simulink model "complete_controller_unorganized"  (R2023a)
settings: Solver=FixedStepAuto  StartTime=0.0  StopTime=inf  FixedStep=0.01  RelTol=1e-3
model workspace (MAT data in the model file):
  SL_ROS_VariableLengthArrays_MaxSizes.CommonInfo.ArrayTruncateAction = 'EmitWarning'
  SL_ROS_VariableLengthArrays_MaxSizes.MsgTypeMap = containers.Map
  SL_ROS_VariableLengthArrays_MaxSizes.MsgTypeMap.serialization.keys = {'diagnostic_msgs/DiagnosticArray', 'diagnostic_msgs/DiagnosticStatus', 'std_msgs/Float32MultiArray', 'std_msgs/Int32MultiArray'}
  SL_ROS_VariableLengthArrays_MaxSizes.MsgTypeMap.serialization.values{1}.PropertyName = 'status'
  SL_ROS_VariableLengthArrays_MaxSizes.MsgTypeMap.serialization.values{1}.DataType = 'diagnostic_msgs/DiagnosticStatus'
  SL_ROS_VariableLengthArrays_MaxSizes.MsgTypeMap.serialization.values{1}.MaxLength = 2
  SL_ROS_VariableLengthArrays_MaxSizes.MsgTypeMap.serialization.values{2}(1).PropertyName = 'hardware_id'
  SL_ROS_VariableLengthArrays_MaxSizes.MsgTypeMap.serialization.values{2}(1).DataType = 'uint8'
  SL_ROS_VariableLengthArrays_MaxSizes.MsgTypeMap.serialization.values{2}(1).MaxLength = 128
  SL_ROS_VariableLengthArrays_MaxSizes.MsgTypeMap.serialization.values{2}(2).PropertyName = 'message'
  SL_ROS_VariableLengthArrays_MaxSizes.MsgTypeMap.serialization.values{2}(2).DataType = 'uint8'
  SL_ROS_VariableLengthArrays_MaxSizes.MsgTypeMap.serialization.values{2}(2).MaxLength = 128
  SL_ROS_VariableLengthArrays_MaxSizes.MsgTypeMap.serialization.values{2}(3).PropertyName = 'name'
  SL_ROS_VariableLengthArrays_MaxSizes.MsgTypeMap.serialization.values{2}(3).DataType = 'uint8'
  SL_ROS_VariableLengthArrays_MaxSizes.MsgTypeMap.serialization.values{2}(3).MaxLength = 128
  SL_ROS_VariableLengthArrays_MaxSizes.MsgTypeMap.serialization.values{2}(4).PropertyName = 'values'
  SL_ROS_VariableLengthArrays_MaxSizes.MsgTypeMap.serialization.values{2}(4).DataType = 'diagnostic_msgs/KeyValue'
  SL_ROS_VariableLengthArrays_MaxSizes.MsgTypeMap.serialization.values{2}(4).MaxLength = 8
  SL_ROS_VariableLengthArrays_MaxSizes.MsgTypeMap.serialization.values{3}.PropertyName = 'data'
  SL_ROS_VariableLengthArrays_MaxSizes.MsgTypeMap.serialization.values{3}.DataType = 'single'
  SL_ROS_VariableLengthArrays_MaxSizes.MsgTypeMap.serialization.values{3}.MaxLength = 8
  SL_ROS_VariableLengthArrays_MaxSizes.MsgTypeMap.serialization.values{4}.PropertyName = 'data'
  SL_ROS_VariableLengthArrays_MaxSizes.MsgTypeMap.serialization.values{4}.DataType = 'int32'
  SL_ROS_VariableLengthArrays_MaxSizes.MsgTypeMap.serialization.values{4}.MaxLength = 8
  SL_ROS_VariableLengthArrays_MaxSizes.MsgTypeMap.serialization.uniformity = 0
  SL_ROS_VariableLengthArrays_MaxSizes.MsgTypeMap.serialization.keyType = 'char'
  SL_ROS_VariableLengthArrays_MaxSizes.MsgTypeMap.serialization.valueType = 'any'
undefined symbols (not defined in the file): angular, Btrigger_boost, DAapply_nudges, DAdesired_pose, DAff_body_force, DAsolver_weights, Djoy_R_X, Dreverse_throttle, Dthrottle, Iangular_mode, Ilinear_mode, linear
libraries: ros2lib x78
(part 1 of 3)
settings Model: Creator=hollis  LastModifiedBy=john
settings OptimizationCC: DefaultParameterBehavior=Inlined  GainParamInheritBuiltInType=on  UseFloatMulNetSlope=on  InlineInvariantSignals=on  EnhancedBackFolding=on  PassReuseOutputArgsAs=Individual arguments  ZeroExternalMemoryAtStartup=off  ZeroInternalMemoryAtStartup=off  EfficientFloat2IntCast=on  MaxStackSize=64  OptimizeBlockOrder=speed  DifferentSizesBufferReuse=on  OptimizationCustomize=off  EfficientTunableParamExpr=on
settings DebuggingCC: ParameterTunabilityLossMsg=error  UnderSpecifiedDimensionMsg=warning
settings HardwareCC: ProdBitPerLong=64  ProdLargestAtomicInteger=LongLong  ProdLargestAtomicFloat=Double  ProdLongLongMode=on  ProdHWDeviceType=ARM Compatible->ARM 64-bit (LP64)
settings SFSimCC: SimUserSources=complete_system/send_thruster_cmd_canbus.c  SimTargetLang=C++
settings RTWCC: Description=Embedded Coder  SystemTargetFile=ert.tlc  HardwareBoard=Robot Operating System 2 (ROS 2)  TLCOptions="-aInlineSetEventsForThisBaseRateFcn=TLC_FALSE -aSuppressMultiTaskScheduler=TLC_FALSE  -aRateBasedStepFcn=0"  TemplateMakefile=ert_default_tmf  CustomSource=complete_system/send_thruster_cmd_canbus.c  Toolchain=Colcon Tools  BuildConfiguration=Faster Runs  TargetLang=C++
settings CodeAppCC: ForceParamTrailComments=on  IgnoreCustomStorageClasses=off  OperatorAnnotations=on  SimulinkDataObjDesc=on  SFDataObjDesc=on  InsertBlockDesc=on
settings ERTTargetCC: TargetLangStandard=C++11 (ISO)  CodeInterfacePackaging=C++ class  SupportVariableSizeSignals=on  InlinedParameterPlacement=NonHierarchical  RootIOFormat=Structure reference

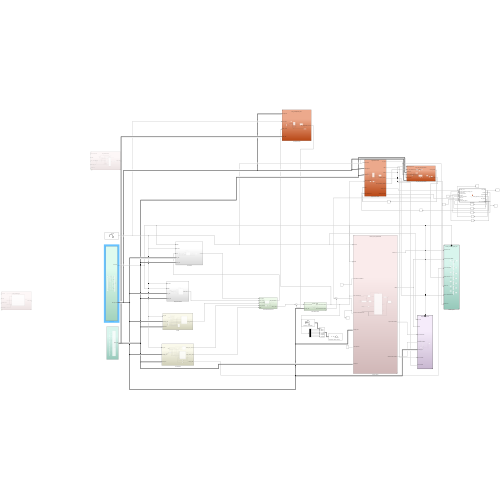
[thumbnail: Simulink's stored preview of the top-level diagram]
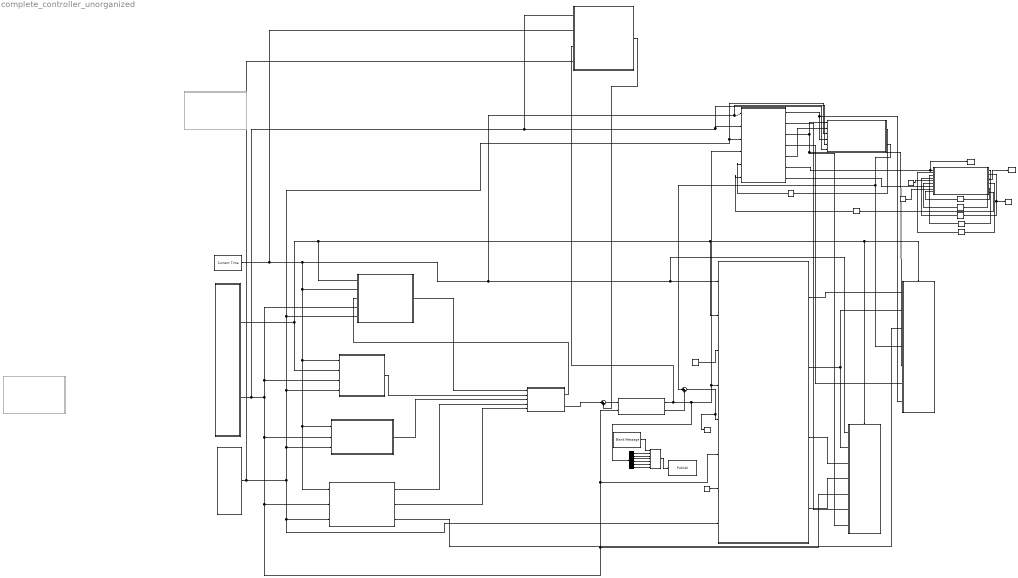
== system complete_controller_unorganized ==
  Applied Force Scale : Subsystem  ReferencedSubsystem=AppliedForceScale
  Auto_FF_Scale_Processor : Subsystem  ReferencedSubsystem=Auto_FF_Scale_Processor
  Blank Message : ros2lib/Blank Message  messageClass=Message  entityType=geometry_msgs/Twist  messageType=geometry_msgs/Twist  SampleTime=inf
  Bus Assignment : BusAssignment  AssignedSignals=linear.x,linear.y,linear.z,angular.x,angular.y,angular.z
  Constant : Constant
  Constant1 : Constant  Value=.005
  Constant2 : Constant  Value=15000
  Constant3 : Constant  Value=[0,0,0]
  Control Mask Management : Subsystem
  Control Mode Mask : Subsystem  ReferencedSubsystem=Disable_Gains
  Current Time : ros2lib/Current Time  OutputFormat=double  SampleTime=-1  ModelName=complete_controller
  Demux : Demux  Outputs=6
  Drag Compensator : Subsystem  ReferencedSubsystem=Drag_Compensator_mk1
  Memory : Memory  InitialCondition=false
  Memory1 : Memory  InitialCondition=[0;0;0]
  Memory2 : Memory
  Memory3 : Memory  InitialCondition=[0;0;0;0;0;0]
  Memory4 : Memory
  Memory5 : Memory
  Memory6 : Memory  InitialCondition=false
  PID Control2 : Subsystem
  Publish : ros2lib/Publish  topicSource=Specify your own  topic=/talos/controller_debug_wrench  messageType=geometry_msgs/Twist  QOSHistory=Keep last  QOSDepth=1  QOSReliability=Reliable  QOSDurability=Volatile
  Publish System : Subsystem  ReferencedSubsystem=Publish_Control_System_Out
  Record : Record  FileSettingsInternal="{\"entries\":[{\"content\":{\"excelSettings\":{\"content\":{},\"type\":\"Streamout.ExcelSettings\"}},\"type\":\"Streamout.FileSettingStorage\",\"uuid\":\"\"}],\"packageUris\":[\"http:\\/\\/schema.mathworks.com\\/mf0\\/streamout_blocks\\/R2020a\"],\"version\":\"1.0\"}"  Layout=[1 1]  SignalsInternal="{\"entries\":[{\"content\":{\"signals\":[{\"content\":{\"blockPath\":[],\"dimensions\":[6,1],\"domain\":\"\",\"hasChildren\":true,\"lineColor\":\"#4dbeee\",\"port\":1,\"signalID\":48,\"signalName\":\"com learner:2\"},\"type\":\"RecordBlkView.Signal\",\"uuid\":\"\"},{\"content\":{\"blockPath\":[],\"channel\":[1,1],\"dimensions\":[6,1],\"domain\":\"\",\"lineColor\":\"#ff13a6\",\"parentID\":48,\"port\":1,\"signalID\":49,\"signalName\":\"com learner:2\"},\"type\":\"RecordBlkView.Signal\",\"uuid\":\"\"}]},\"type\":\"RecordBlkView.InputSignals\",\"uuid\":\"\"}],\"packageUris\":[\"http:\\/\\/schema.mathworks.com\\/mf0\\/streamout_blocks\\/R2020a\"],\"version\":\"1.0\"}"  VisualizationBindings="{\"sparklinesplugin\":{\"info\":[{\"bindingParametersList\":[],\"subplotID\":1}]}}"
  Record1 : Record  FileSettingsInternal="{\"entries\":[{\"content\":{\"excelSettings\":{\"content\":{},\"type\":\"Streamout.ExcelSettings\"}},\"type\":\"Streamout.FileSettingStorage\",\"uuid\":\"\"}],\"packageUris\":[\"http:\\/\\/schema.mathworks.com\\/mf0\\/streamout_blocks\\/R2020a\"],\"version\":\"1.0\"}"  Layout=[1 1]  SignalsInternal="{\"entries\":[{\"content\":{\"signals\":[{\"content\":{\"blockPath\":[],\"dimensions\":[6,1],\"domain\":\"\",\"hasChildren\":true,\"lineColor\":\"#139fff\",\"port\":1,\"signalID\":36,\"signalName\":\"Applied Force Scale:6\"},\"type\":\"RecordBlkView.Signal\",\"uuid\":\"\"},{\"content\":{\"blockPath\":[],\"channel\":[1,1],\"dimensions\":[6,1],\"domain\":\"\",\"lineColor\":\"#22b573\",\"parentID\":36,\"port\":1,\"signalID\":37,\"signalName\":\"Applied Force Scale:6\"},\"type\":\"RecordBlkView.Signal\",\"uuid\":\"\"}]},\"type\":\"RecordBlkView.InputSignals\",\"uuid\":\"\"}],\"packageUris\":[\"http:\\/\\/schema.mathworks.com\\/mf0\\/streamout_blocks\\/R2020a\"],\"version\":\"1.0\"}"  VisualizationBindings="{\"sparklinesplugin\":{\"info\":[{\"bindingParametersList\":[],\"subplotID\":1}]}}"
  Record2 : Record  FileSettingsInternal="{\"entries\":[{\"content\":{\"excelSettings\":{\"content\":{},\"type\":\"Streamout.ExcelSettings\"}},\"type\":\"Streamout.FileSettingStorage\",\"uuid\":\"\"}],\"packageUris\":[\"http:\\/\\/schema.mathworks.com\\/mf0\\/streamout_blocks\\/R2020a\"],\"version\":\"1.0\"}"  SignalsInternal="{\"entries\":[{\"content\":{\"signals\":[{\"content\":{\"blockPath\":[],\"dimensions\":[3,1],\"domain\":\"\",\"hasChildren\":true,\"lineColor\":\"#b746ff\",\"port\":1,\"signalID\":25,\"signalName\":\"com learner:3\"},\"type\":\"RecordBlkView.Signal\",\"uuid\":\"\"},{\"content\":{\"blockPath\":[],\"channel\":[1,1],\"dimensions\":[3,1],\"domain\":\"\",\"lineColor\":\"#d95319\",\"parentID\":25,\"plots\":[1],\"port\":1,\"signalID\":26,\"signalName\":\"com learner:3\"},\"type\":\"RecordBlkView.Signal\",\"uuid\":\"\"},{\"content\":{\"blockPath\":[],\"channel\":[2,1],\"dimensions\":[3,1],\"domain\":\"\",\"lineColor\":\"#22b573\",\"parentID\":25,\"plots\":[1],\"port\":1,\"signalID\":27,\"signalName\":\"com learner:3\"},\"type\":\"RecordBlkView.Signal\",\"uuid\":\"\"},{\"content\":{\"blockPath\":[],\"channel\":[3,1],\"dimensions\":[3,1],\"domain\":\"\",\"lineColor\":\"#0072bd\",\"parentID\":25,\"plots\":[1],\"port\":1,\"signalID\":28,\"signalName\":\"com learner:3\"},\"type\":\"RecordBlkView.Signal\",\"uuid\":\"\"}]},\"type\":\"RecordBlkView.InputSignals\",\"uuid\":\"\"}],\"packageUris\":[\"http:\\/\\/schema.mathworks.com\\/mf0\\/streamout_blocks\\/R2020a\"],\"version\":\"1.0\"}"  VisualizationBindings="{\"sparklinesplugin\":{\"info\":[{\"bindingParametersList\":[],\"subplotID\":1}]}}"
  Record3 : Record  FileSettingsInternal="{\"entries\":[{\"content\":{\"excelSettings\":{\"content\":{},\"type\":\"Streamout.ExcelSettings\"}},\"type\":\"Streamout.FileSettingStorage\",\"uuid\":\"\"}],\"packageUris\":[\"http:\\/\\/schema.mathworks.com\\/mf0\\/streamout_blocks\\/R2020a\"],\"version\":\"1.0\"}"  Layout=[1 1]  SignalsInternal="{\"entries\":[{\"content\":{\"signals\":[{\"content\":{\"blockPath\":[],\"dimensions\":[6],\"domain\":\"\",\"hasChildren\":true,\"lineColor\":\"#ff13a6\",\"port\":1,\"signalID\":8,\"signalName\":\"Sum\"},\"type\":\"RecordBlkView.Signal\",\"uuid\":\"\"},{\"content\":{\"blockPath\":[],\"channel\":[1],\"dimensions\":[6],\"domain\":\"\",\"lineColor\":\"#64d413\",\"parentID\":8,\"plots\":[1],\"port\":1,\"signalID\":9,\"signalName\":\"Sum\"},\"type\":\"RecordBlkView.Signal\",\"uuid\":\"\"},{\"content\":{\"blockPath\":[],\"channel\":[2],\"dimensions\":[6],\"domain\":\"\",\"lineColor\":\"#0072bd\",\"parentID\":8,\"plots\":[1],\"port\":1,\"signalID\":10,\"signalName\":\"Sum\"},\"type\":\"RecordBlkView.Signal\",\"uuid\":\"\"},{\"content\":{\"blockPath\":[],\"channel\":[3],\"dimensions\":[6],\"domain\":\"\",\"lineColor\":\"#d95319\",\"parentID\":8,\"plots\":[1],\"port\":1,\"signalID\":11,\"signalName\":\"Sum\"},\"type\":\"RecordBlkView.Signal\",\"uuid\":\"\"},{\"content\":{\"blockPath\":[],\"channel\":[4],\"dimensions\":[6],\"domain\":\"\",\"lineColor\":\"#edb120\",\"parentID\":8,\"plots\":[1],\"port\":1,\"signalID\":12,\"signalName\":\"Sum\"},\"type\":\"RecordBlkView.Signal\",\"uuid\":\"\"},{\"content\":{\"blockPath\":[],\"channel\":[5],\"dimensions\":[6],\"domain\":\"\",\"lineColor\":\"#7e2f8e\",\"parentID\":8,\"plots\":[1],\"port\":1,\"signalID\":13,\"signalName\":\"Sum\"},\"type\":\"RecordBlkView.Signal\",\"uuid\":\"\"},{\"content\":{\"blockPath\":[],\"channel\":[6],\"dimensions\":[6],\"domain\":\"\",\"lineColor\":\"#77ac30\",\"parentID\":8,\"plots\":[1],\"port\":1,\"signalID\":14,\"signalName\":\"Sum\"},\"type\":\"RecordBlkView.Signal\",\"uuid\":\"\"}]},\"type\":\"RecordBlkView.InputSignals\",\"uuid\":\"\"}],\"packageUris\":[\"http:\\/\\/schema.mathworks.com\\/mf0\\/streamout_blocks\\/R2020a\"],\"version\":\"1.0\"}"  VisualizationBindings="{\"sparklinesplugin\":{\"info\":[{\"bindingParametersList\":[],\"subplotID\":1}]}}"
  Sliding Mode Control : Subsystem
  Stunt Controller : Subsystem
  Subsystem : Subsystem
  Subsystem Reference : Subsystem  Commented=on  ReferencedSubsystem=PID_Mathmatical
      settings: PortSchema="{\"entries\":[{\"content\":{\"sides\":[{\"content\":{\"connectorIds\":[\"In2\",\"In1\",\"In3\",\"In5\",\"In4\"]},\"type\":\"ConnectorPlacement.EquallySpacedRectSide\",\"uuid\":\"8e3db528-7e61-4c43-b00e-51bc92e38ec5\"},{\"content\":{\"connectorIds\":[\"Out1\"],\"side\":\"RIGHT\"},\"type\":\"ConnectorPlacement.EquallySpacedRectSide\",\"uuid\":\"f86917d4-f680-48e1-82f7-3e38b9d3dfda\"},{\"content\":{\"side\":\"TOP\"},\"type\":\"ConnectorPlacement.EquallySpacedRectSide\",\"uuid\":\"74f2307a-7295-42c0-bea9-7bac6b4d27cf\"}]},\"type\":\"ConnectorPlacement.EquallySpacedConnector\",\"uuid\":\"49652a12-83c7-468f-bb5a-320f9b02978b\"}],\"packageUris\":[\"http://schema.mathworks.com/mf0/Connector/R2020b\"],\"version\":\"1.0\"}"
  Subsystem Reference1 : Subsystem  Commented=on  ReferencedSubsystem=SMC_mathmatical
      settings: PortSchema="{\"entries\":[{\"content\":{\"sides\":[{\"content\":{\"connectorIds\":[\"In1\",\"In2\",\"In4\",\"In3\"]},\"type\":\"ConnectorPlacement.EquallySpacedRectSide\",\"uuid\":\"d99f1ec8-d0dd-4591-8b28-a91bcf98a65e\"},{\"content\":{\"connectorIds\":[\"Out1\"],\"side\":\"RIGHT\"},\"type\":\"ConnectorPlacement.EquallySpacedRectSide\",\"uuid\":\"f211976d-83c1-4660-96a4-4139d6a3eac5\"},{\"content\":{\"side\":\"TOP\"},\"type\":\"ConnectorPlacement.EquallySpacedRectSide\",\"uuid\":\"9c887152-ce22-4e53-9dff-b8a725742b50\"}]},\"type\":\"ConnectorPlacement.EquallySpacedConnector\",\"uuid\":\"34693693-7ca6-4fc8-a99f-a057e134d206\"}],\"packageUris\":[\"http://schema.mathworks.com/mf0/Connector/R2020b\"],\"version\":\"1.0\"}"
  Subsystem Reference3 : Subsystem  ReferencedSubsystem=Diagnostic_Reporter
  Subsystem1 : Subsystem
  Sum : Sum  Inputs=|++
  Sum1 : Sum  Inputs=|++
  TeleOp : Subsystem
  Thruster Solver : Subsystem  ReferencedSubsystem=Thruster_Solver_Mathmatical
      settings: PortSchema="{\"entries\":[{\"content\":{\"sides\":[{\"content\":{\"connectorIds\":[\"In1\",\"In2\",\"In3\",\"In4\",\"In5\",\"In7\",\"In8\",\"In6\"]},\"type\":\"ConnectorPlacement.EquallySpacedRectSide\",\"uuid\":\"7443c28d-8cee-4065-b63f-8039eaddf426\"},{\"content\":{\"connectorIds\":[\"Out1\",\"Out2\",\"Out3\",\"Out4\"],\"side\":\"RIGHT\"},\"type\":\"ConnectorPlacement.EquallySpacedRectSide\",\"uuid\":\"625b2eba-64d9-4ade-9893-8e78eb613954\"},{\"content\":{\"side\":\"TOP\"},\"type\":\"ConnectorPlacement.EquallySpacedRectSide\",\"uuid\":\"e2df6dfc-d16d-465d-896d-535154799a49\"}]},\"type\":\"ConnectorPlacement.EquallySpacedConnector\",\"uuid\":\"d998c598-ebfe-49fc-a537-223cf8fafed3\"}],\"packageUris\":[\"http://schema.mathworks.com/mf0/Connector/R2020b\"],\"version\":\"1.0\"}"
  com learner : MATLAB Function  TreatAsAtomicUnit=on
  wires:
  Current Time/1 -> Drag Compensator/2, PID Control2/2(ROS Time), TeleOp/1(ros_time), Stunt Controller/1(ros_time), Sliding Mode Control/1(ROS Time), Auto_FF_Scale_Processor/5, Applied Force Scale/1, Subsystem Reference3/1, Thruster Solver/1
  Thruster Solver/1 -> Publish System/1
  Thruster Solver/2 -> Subsystem Reference3/2, Publish System/2
  Constant/1 -> Thruster Solver/3
  Thruster Solver/3 -> Subsystem Reference3/3
  Thruster Solver/4 -> Subsystem Reference3/4
  PID Control2/1(control) -> Control Mask Management/1(PID_Control)
  Sliding Mode Control/1(Control Forces) -> Control Mask Management/2(SMC_Control)
  TeleOp/1(teleop_control) -> Control Mask Management/3(Teleop_Control)
  Stunt Controller/1(stunt_active_control) -> Control Mask Management/4(Stunt_Control)
  Stunt Controller/2(control_mode_mask) -> Control Mask Management/5(mask)
  Control Mask Management/1(clear_accumulators) -> PID Control2/3(reset)
  Stunt Controller/3(running_state) -> Publish System/3
  Subsystem1/1(New State) -> Sliding Mode Control/2(Enable), PID Control2/1(Enable), Publish System/Enable, Subsystem Reference3/Enable, Thruster Solver/2
  Subsystem1/2(Message Bus) -> Drag Compensator/1, Auto_FF_Scale_Processor/6, Applied Force Scale/2, PID Control2/4(msg_bus), Sliding Mode Control/3(msg_bus), Subsystem Reference3/5, Control Mode Mask/2, Thruster Solver/7, Stunt Controller/2(message_bus), TeleOp/2(message_bus)
  Subsystem/1(param_bus) -> Drag Compensator/4, Thruster Solver/6, Stunt Controller/3(param_bus), PID Control2/5(param_bus), Auto_FF_Scale_Processor/3, Applied Force Scale/3, Sliding Mode Control/4(param_bus), TeleOp/3(param bus)  "param bus"
  Control Mask Management/2(active_control) -> Sum1/1
  Control Mode Mask/2 -> Sum/2
  Sum/1 -> Record3/1, Thruster Solver/5
  Applied Force Scale/4 -> Publish System/6
  Applied Force Scale/3 -> Subsystem Reference3/7, Publish System/5, Auto_FF_Scale_Processor/1
  Applied Force Scale/1 -> Auto_FF_Scale_Processor/4, Publish System/7
  Auto_FF_Scale_Processor/1 -> Memory/1
  Auto_FF_Scale_Processor/2 -> Publish System/4, Sum/1
  Applied Force Scale/2 -> Subsystem Reference3/6
  Memory/1 -> Applied Force Scale/5
  Applied Force Scale/5 -> Auto_FF_Scale_Processor/2
  Sum1/1 -> Control Mode Mask/1
  Drag Compensator/1 -> Sum1/2
  Blank Message/1 -> Bus Assignment/1
  Bus Assignment/1 -> Publish/1
  Demux/1 -> Bus Assignment/2
  Demux/2 -> Bus Assignment/3
  Demux/3 -> Bus Assignment/4
  Demux/4 -> Bus Assignment/5
  Demux/5 -> Bus Assignment/6
  Demux/6 -> Bus Assignment/7
  Control Mode Mask/1 -> Drag Compensator/3, Demux/1, Applied Force Scale/4, Thruster Solver/4
  Applied Force Scale/6 -> Record1/1, com learner/1(average_error)
  Constant1/1 -> com learner/5(resolution)
  Memory1/1 -> com learner/6(previous_application)
  Memory2/1 -> com learner/9(previous_last_applied)
  com learner/5(last_applied) -> Memory2/1
  Memory3/1 -> com learner/4(previous_rewards)
  com learner/2(rewards) -> Record/1, Memory3/1
  Memory4/1 -> com learner/2(previous_adjustment_average_error)
  com learner/4(latest_adjustment_average_error) -> Memory4/1
  Memory5/1 -> com learner/3(previous_state)
  com learner/1(new_state) -> Memory5/1
  com learner/3(application) -> Record2/1, Memory1/1
  com learner/6(reset_accumulator) -> Memory6/1  "reset_Accumulator"
  Applied Force Scale/7 -> com learner/7(total_time)
  Constant2/1 -> com learner/8(eval_time)
  Memory6/1 -> Applied Force Scale/6
  Constant3/1 -> Thruster Solver/8

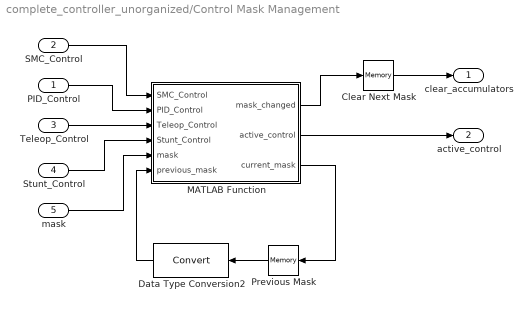
== system complete_controller_unorganized/Control Mask Management ==
  PID_Control : Inport
  SMC_Control : Inport  Port=2
  Teleop_Control : Inport  Port=3
  Stunt_Control : Inport  Port=4
  mask : Inport  Port=5
  Clear Next Mask : Memory
  Data Type Conversion2 : DataTypeConversion  SaturateOnIntegerOverflow=off  RndMeth=Floor
  MATLAB Function : MATLAB Function  TreatAsAtomicUnit=on
  Previous Mask : Memory  InitialCondition=[0,0,0,0,0,0]
  clear_accumulators : Outport
  active_control : Outport  Port=2
  wires:
  Previous Mask/1 -> Data Type Conversion2/1
  SMC_Control/1 -> MATLAB Function/1(SMC_Control)
  PID_Control/1 -> MATLAB Function/2(PID_Control)
  MATLAB Function/2(active_control) -> active_control/1
  Stunt_Control/1 -> MATLAB Function/4(Stunt_Control)
  Data Type Conversion2/1 -> MATLAB Function/6(previous_mask)
  Teleop_Control/1 -> MATLAB Function/3(Teleop_Control)
  MATLAB Function/1(mask_changed) -> Clear Next Mask/1
  mask/1 -> MATLAB Function/5(mask)
  MATLAB Function/3(current_mask) -> Previous Mask/1
  Clear Next Mask/1 -> clear_accumulators/1

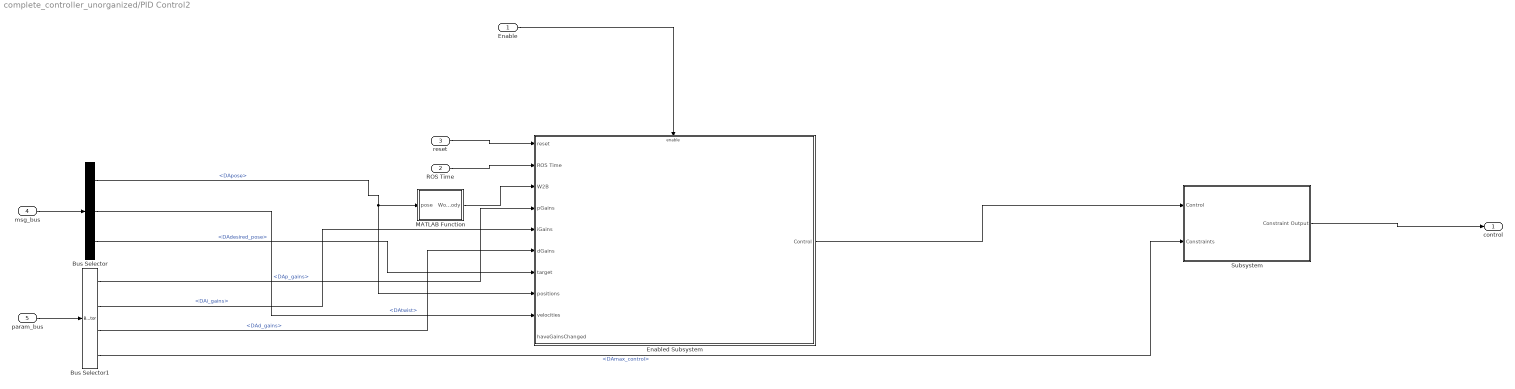
== system complete_controller_unorganized/PID Control2 ==
  Enable : Inport
  ROS Time : Inport  Port=2
  reset : Inport  Port=3
  msg_bus : Inport  Port=4
  param_bus : Inport  Port=5
  Bus Selector : BusSelector  OutputSignals=current_state.DApose,current_state.DAtwist,desired_pose.DAdesired_pose
  Bus Selector1 : BusSelector  OutputSignals=DAp_gains,DAi_gains,DAd_gains,DAmax_control
  Enabled Subsystem : Subsystem  TreatAsAtomicUnit=on
  MATLAB Function : MATLAB Function  TreatAsAtomicUnit=on
  Subsystem : Subsystem
  control : Outport
  wires:
  param_bus/1 -> Bus Selector1/1
  Enable/1 -> Enabled Subsystem/Enable
  reset/1 -> Enabled Subsystem/1(reset)
  ROS Time/1 -> Enabled Subsystem/2(ROS Time)
  Bus Selector1/1 -> Enabled Subsystem/4(pGains)  "<DAp_gains>"
  Bus Selector1/2 -> Enabled Subsystem/5(iGains)  "<DAi_gains>"
  Bus Selector1/3 -> Enabled Subsystem/6(dGains)  "<DAd_gains>"
  Bus Selector1/4 -> Subsystem/2(Constraints)  "<DAmax_control>"
  msg_bus/1 -> Bus Selector/1
  Bus Selector/1 -> MATLAB Function/1(pose), Enabled Subsystem/8(positions)  "<DApose>"
  Bus Selector/2 -> Enabled Subsystem/9(velocities)  "<DAtwist>"
  Bus Selector/3 -> Enabled Subsystem/7(target)  "<DAdesired_pose>"
  MATLAB Function/1(World2Body) -> Enabled Subsystem/3(W2B)
  Subsystem/1(Constraint Output) -> control/1
  Enabled Subsystem/1(Control) -> Subsystem/1(Control)

== system complete_controller_unorganized/Sliding Mode Control ==
  ROS Time : Inport
  Enable : Inport  Port=2
  msg_bus : Inport  Port=3
  param_bus : Inport  Port=4
  Bus Selector : BusSelector  OutputSignals=current_state.DApose,current_state.DAtwist,desired_pose.DAdesired_pose
  Subsystem : Subsystem
  Control Forces : Outport
  wires:
  msg_bus/1 -> Bus Selector/1
  ROS Time/1 -> Subsystem/1(ROS Time)
  Enable/1 -> Subsystem/Enable
  Bus Selector/1 -> Subsystem/2(Current Positions)  "<DApose>"
  Bus Selector/2 -> Subsystem/3(World Velocities)  "<DAtwist>"
  Bus Selector/3 -> Subsystem/4(Target Positions)  "<DAdesired_pose>"
  param_bus/1 -> Subsystem/5(param_bus)
  Subsystem/1(Control Forces) -> Control Forces/1

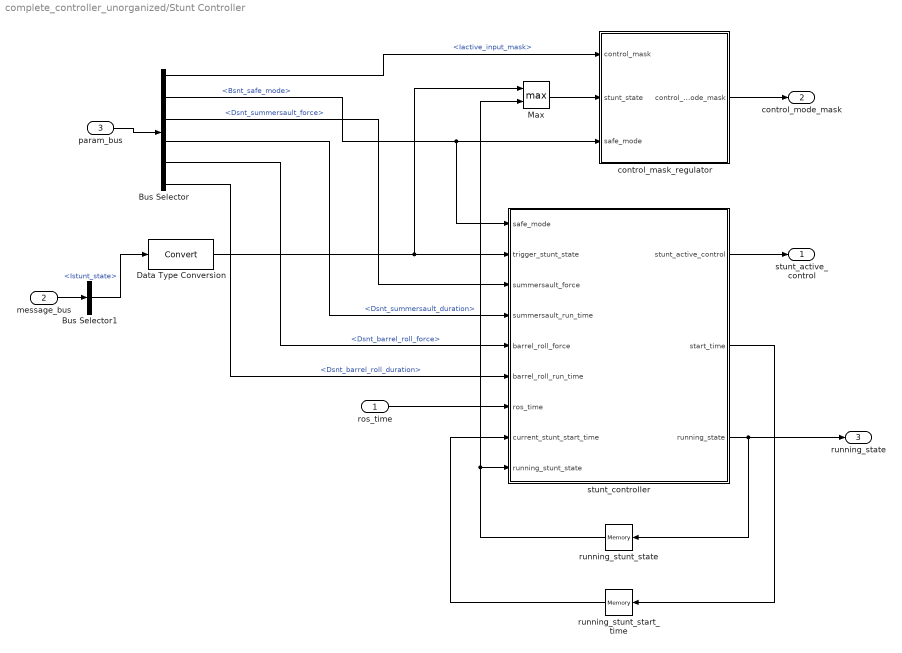
== system complete_controller_unorganized/Stunt Controller ==
  ros_time : Inport
  message_bus : Inport  Port=2
  param_bus : Inport  Port=3
  Bus Selector : BusSelector  OutputSignals=Iactive_input_mask,Bsnt_safe_mode,Dsnt_summersault_force,Dsnt_summersault_duration,Dsnt_barrel_roll_force,Dsnt_barrel_roll_duration
  Bus Selector1 : BusSelector  OutputSignals=Istunt_state
  Data Type Conversion : DataTypeConversion  SaturateOnIntegerOverflow=off  RndMeth=Floor
  Max : MinMax  Function=max  Inputs=2
  control_mask_regulator : MATLAB Function  TreatAsAtomicUnit=on
  running_stunt_start_time : Memory
  running_stunt_state : Memory
  stunt_controller : MATLAB Function  TreatAsAtomicUnit=on
  stunt_active_control : Outport
  control_mode_mask : Outport  Port=2
  running_state : Outport  Port=3
  wires:
  control_mask_regulator/1(control_mode_mask) -> control_mode_mask/1
  stunt_controller/3(running_state) -> running_stunt_state/1, running_state/1
  stunt_controller/2(start_time) -> running_stunt_start_time/1
  running_stunt_state/1 -> stunt_controller/9(running_stunt_state), Max/2
  running_stunt_start_time/1 -> stunt_controller/8(current_stunt_start_time)
  stunt_controller/1(stunt_active_control) -> stunt_active_control/1
  Bus Selector/3 -> stunt_controller/3(summersault_force)  "<Dsnt_summersault_force>"
  Bus Selector/4 -> stunt_controller/4(summersault_run_time)  "<Dsnt_summersault_duration>"
  ros_time/1 -> stunt_controller/7(ros_time)
  Bus Selector/6 -> stunt_controller/6(barrel_roll_run_time)  "<Dsnt_barrel_roll_duration>"
  Bus Selector/5 -> stunt_controller/5(barrel_roll_force)  "<Dsnt_barrel_roll_force>"
  Max/1 -> control_mask_regulator/2(stunt_state)
  param_bus/1 -> Bus Selector/1
  Bus Selector/2 -> stunt_controller/1(safe_mode), control_mask_regulator/3(safe_mode)  "<Bsnt_safe_mode>"
  Bus Selector/1 -> control_mask_regulator/1(control_mask)  "<Iactive_input_mask>"
  message_bus/1 -> Bus Selector1/1
  Bus Selector1/1 -> Data Type Conversion/1  "<Istunt_state>"
  Data Type Conversion/1 -> Max/1, stunt_controller/2(trigger_stunt_state)
